simulink model "soal2_2"  (R2023b)
settings: Solver=ode4  StartTime=0.0  StopTime=30  FixedStep=0.01  RelTol=1e-3
InitFcn:
  | Ts = 0.01;
settings Model: Creator=amir  LastModifiedBy=amir

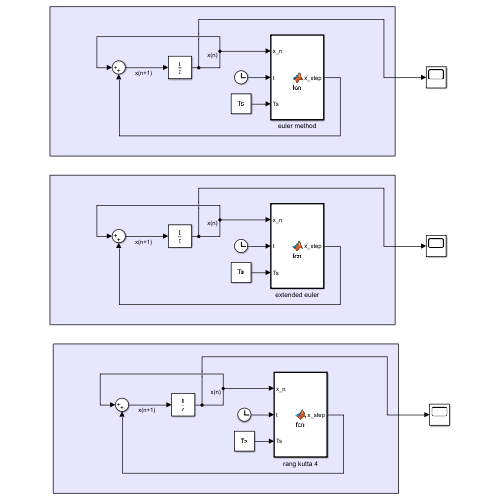
[thumbnail: Simulink's stored preview of the top-level diagram]
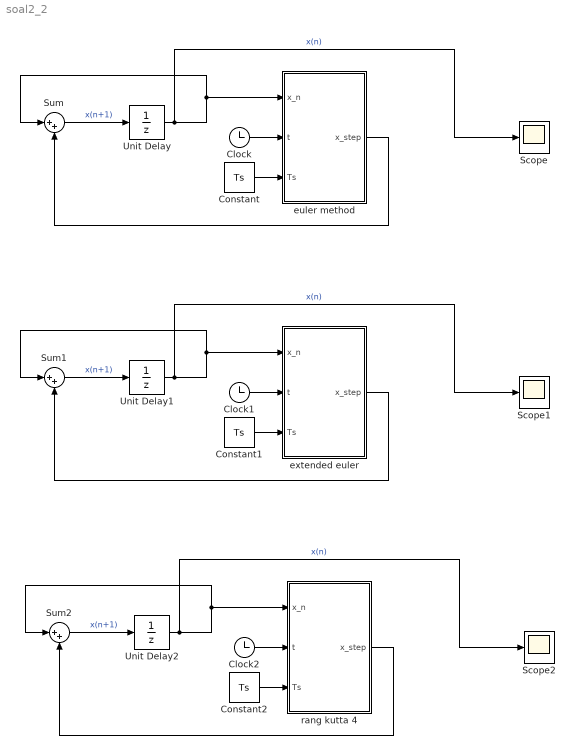
== system soal2_2 ==
  Clock : Clock
  Clock1 : Clock
  Clock2 : Clock
  Constant : Constant  Value=Ts
  Constant1 : Constant  Value=Ts
  Constant2 : Constant  Value=Ts
  Scope : Scope
  Scope1 : Scope
  Scope2 : Scope
  Sum : Sum  Inputs=|++
  Sum1 : Sum  Inputs=|++
  Sum2 : Sum  Inputs=|++
  Unit Delay : UnitDelay  InitialCondition=[0;0]  SampleTime=-1  HasFrameUpgradeWarning=on
  Unit Delay1 : UnitDelay  InitialCondition=[0;0]  SampleTime=-1  HasFrameUpgradeWarning=on
  Unit Delay2 : UnitDelay  InitialCondition=[0;0]  SampleTime=-1  HasFrameUpgradeWarning=on
  euler method : MATLAB Function  TreatAsAtomicUnit=on
  extended euler : MATLAB Function  TreatAsAtomicUnit=on
  rang kutta 4 : MATLAB Function  TreatAsAtomicUnit=on
  wires:
  Sum/1 -> Unit Delay/1  "x(n+1)"
  Unit Delay/1 -> Scope/1, Sum/1, euler method/1(x_n)  "x(n)"
  Clock/1 -> euler method/2(t)
  Constant/1 -> euler method/3(Ts)
  euler method/1(x_step) -> Sum/2
  extended euler/1(x_step) -> Sum1/2
  Clock1/1 -> extended euler/2(t)
  Constant1/1 -> extended euler/3(Ts)
  Unit Delay1/1 -> Scope1/1, Sum1/1, extended euler/1(x_n)  "x(n)"
  Sum1/1 -> Unit Delay1/1  "x(n+1)"
  rang kutta 4/1(x_step) -> Sum2/2
  Clock2/1 -> rang kutta 4/2(t)
  Constant2/1 -> rang kutta 4/3(Ts)
  Unit Delay2/1 -> Scope2/1, Sum2/1, rang kutta 4/1(x_n)  "x(n)"
  Sum2/1 -> Unit Delay2/1  "x(n+1)"

== matlab function soal2_2/euler method ==
  data: x_n input; x_step output; t input; Ts input
function x_step = fcn(x_n, t, Ts)

x_step = [x_n(1,1)*x_n(2,1) - 0.3 * cos(2 * pi * t);
          -x_n(2,1) + x_n(1,1)] * Ts;

== matlab function soal2_2/rang kutta 4 ==
  data: x_n input; x_step output; t input; Ts input
function x_step = fcn(x_n, t, Ts)

dx1 = [x_n(1,1)*x_n(2,1) - 0.3 * cos(2 * pi * t);
          -x_n(2,1) + x_n(1,1)] * Ts;

dx2 = [(x_n(1,1)+dx1(1,1)/2)*(x_n(2,1)+dx1(2,1)/2) - 0.3 * cos(2 * pi * t);
          -(x_n(2,1)+dx1(2,1)/2) + (x_n(1,1)+dx1(1,1)/2)] * Ts;

dx3 = [(x_n(1,1)+dx2(1,1)/2)*(x_n(2,1)+dx2(2,1)/2) - 0.3 * cos(2 * pi * t);
          -(x_n(2,1)+dx2(2,1)/2) + (x_n(1,1)+dx2(1,1)/2)] * Ts;

dx4 = [(x_n(1,1)+dx3(1,1))*(x_n(2,1)+dx3(2,1)) - 0.3 * cos(2 * pi * t);
          -(x_n(2,1)+dx3(2,1)) + (x_n(1,1)+dx3(1,1))] * Ts;
x_step = (1/6) * (dx1 + 2 * dx2 + 2 * dx3 + dx4);

== matlab function soal2_2/extended euler ==
  data: x_n input; x_step output; t input; Ts input
function x_step = fcn(x_n, t, Ts)

dx1 = [x_n(1,1)*x_n(2,1) - 0.3 * cos(2 * pi * t);
          -x_n(2,1) + x_n(1,1)] * Ts;

dx2 = [(x_n(1,1)+dx1(1,1))*(x_n(2,1)+dx1(2,1)) - 0.3 * cos(2 * pi * t);
          -(x_n(2,1)+dx1(2,1)) + (x_n(1,1)+dx1(1,1))] * Ts;
x_step = 0.5 * (dx1 + dx2);
